simulink model "DAB Converters ude"  (R2022a)
settings: Solver=VariableStepAuto  StartTime=0.0  StopTime=0.7  RelTol=1e-3
libraries: spsMosfetLib x16, spsSeriesRLCBranchLib x8, spsCurrentMeasurementLib x4, spsLinearTransformerLib x4, simulink_extras x4, spsSawtoothGeneratorLib x4, spsVoltageMeasurementLib x4, spspowerguiLib x3, spsControlledVoltageSourceLib x2, spsIdealSwitchLib x2, slpidlib x1
settings Model: Creator=shuai  LastModifiedBy=shuai

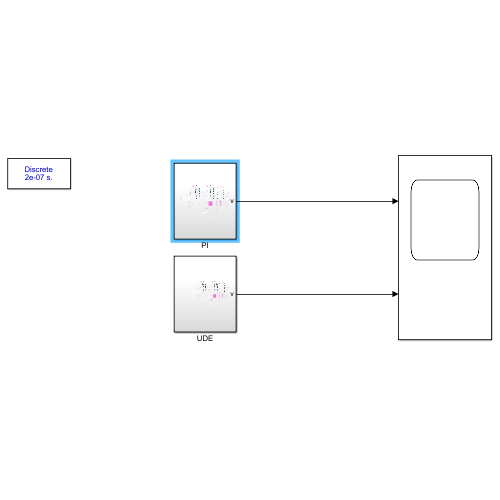
[thumbnail: Simulink's stored preview of the top-level diagram]
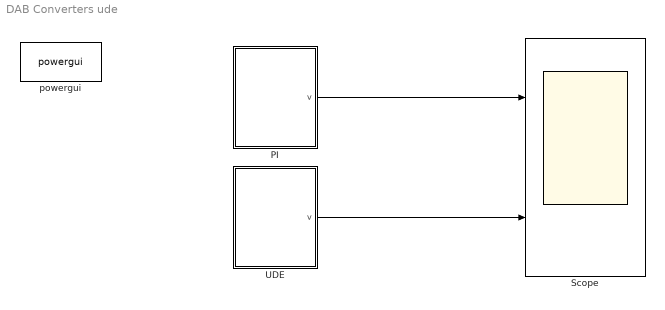
== system DAB Converters ude ==
  PI : Subsystem
  Scope : Scope  NumInputPorts=2
  UDE : Subsystem
  powergui : spspowerguiLib/powergui  Priority=1  SimulationMode=Discrete  SampleTime=2e-7  frequency=60  Iterations=50  frequencyindice=0  Pbase=100e6  ErrMax=1e-4  UnitsV=kV  UnitsW=MW  buscounter=0  FunctionMessages=off  echomessages=off  EnableUseOfTLC=off  CurrentSourceSwitches=off  DisableSnubberDevices=off  DisableRonSwitches=off  DisableVfSwitches=off  DisplayEquations=off  AutomaticDiscreteSolvers=off  SolverType=Tustin/Backward Euler (TBE)  Interpol=off  ExternalGateDelay=off  methode=off  Ts=100  x0status=blocks  SPID=on  SwTol=0  HookPort=off  NonlinearTolerance=1e-4  nMaxIteration=100  ContinueOnMaxIteration=off  RestoreLinks=warning  ResistiveCurrentMeasurement=off  Frange=[0:2:500]  Ylog=off  Xlog=on  ShowGrid=off  save=off  variable=ZData  structure=0  ZoomFFT=off  StartTime=0.0  cycles=1  DisplayStyle=1  fundamental=60  FreqAxis=off  MaxFrequency=1000  frequencyindicesteady=1  RmsSteady=1  display=off
  wires:
  UDE/1(v) -> Scope/2
  PI/1(v) -> Scope/1

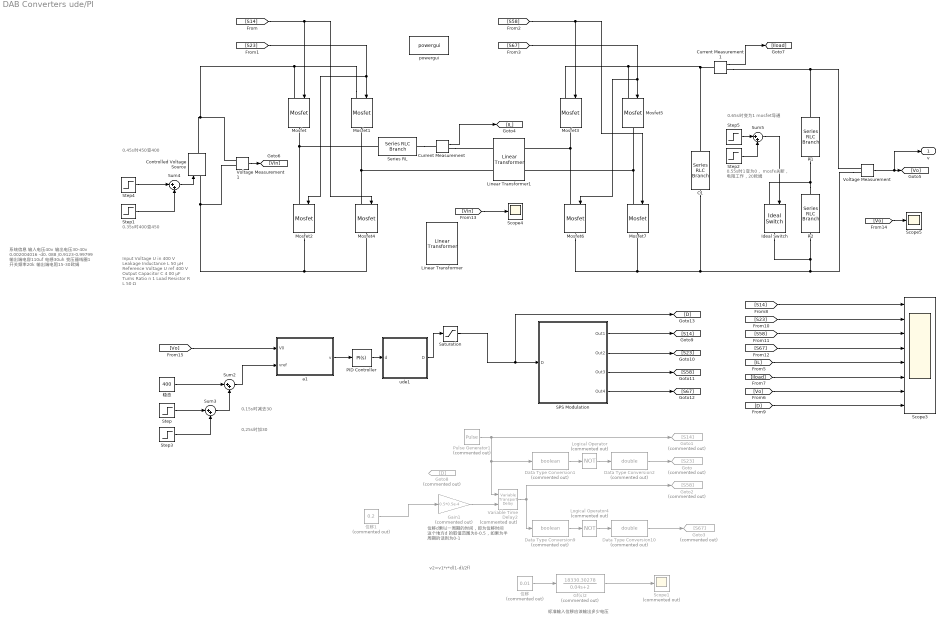
== system DAB Converters ude/PI ==
  note: 0.55s时1变为0，
      | mosfe关断，
      | 电阻工作，20欧姆
  note: 0.65s时变为1 mosfet导通
  note: 0.35s时400变450
  note: 0,15s时减去30
  note: 位移d乘以一周期的时间，即为位移时间
      | 这个地方d 的取值范围为0-0.5，如果为半
      | 周期的话则为0-1
  note: Input Voltage U in 400 V
      | Leakage Inductance L 50 µH
      | Reference Voltage U ref 400 V
      | Output Capacitor C 4 00 µF
      | Turns Ratio n 1
      | Load Resistor R L 50 Ω
  note: v2=v1*r*d(1-d)/2fl
  note: 系统信息
      | 输入电压40v
      | 输出电压30-40v
      | 0.002004016 -d0. 088 /0.9123-0.99799
      | 输出端电容110uf
      | 电感30uh
      | 变压器线圈1
      | 开关频率20k
      | 输出端电阻15-30欧姆
  note: 标准输入位移应该输出多少电压
  note: 0,25s时加30
  note: 0.45s时450变400
  C1 : spsSeriesRLCBranchLib/Series RLC Branch  LConnTagsString=__new0  RConnTagsString=__new0  BranchType=C  Resistance=0.01  Inductance=1e-3  SetiL0=off  InitialCurrent=0  Capacitance=400e-6  Setx0=on  InitialVoltage=0  Measurements=None
  Controlled Voltage Source : spsControlledVoltageSourceLib/Controlled Voltage Source  Initialize=on  Source_Type=DC  Amplitude=0  Phase=0  Frequency=0  Measurements=None
  Current Measurement : spsCurrentMeasurementLib/Current Measurement  PhasorSimulation=off  OutputType=Complex  PSBequivalent=0
  Current Measurement1 : spsCurrentMeasurementLib/Current Measurement  PhasorSimulation=off  OutputType=Complex  PSBequivalent=0
  Data Type Conversion1 : DataTypeConversion  Commented=on  OutDataTypeStr=boolean  SaturateOnIntegerOverflow=off  RndMeth=Floor
  Data Type Conversion10 : DataTypeConversion  Commented=on  OutDataTypeStr=double  SaturateOnIntegerOverflow=off  RndMeth=Floor
  Data Type Conversion2 : DataTypeConversion  Commented=on  OutDataTypeStr=double  SaturateOnIntegerOverflow=off  RndMeth=Floor
  Data Type Conversion9 : DataTypeConversion  Commented=on  OutDataTypeStr=boolean  SaturateOnIntegerOverflow=off  RndMeth=Floor
  Gain1 : Gain  Commented=on  Gain=0.5*0.5e-4
  Gf(s)2 : TransferFcn  Commented=on  Numerator=[18330.30278]  Denominator=[0.04 2]
  Goto : Goto  Commented=on  GotoTag=S23
  Goto1 : Goto  Commented=on  GotoTag=S14
  Goto2 : Goto  Commented=on  GotoTag=S58
  Goto3 : Goto  Commented=on  GotoTag=S67
  Goto8 : Goto  Commented=on  GotoTag=D
  Ideal Switch : spsIdealSwitchLib/Ideal Switch  Ron=0.001  Lon=0  IC=0  Rs=1e5  Cs=inf  Measurements=off
  Linear Transformer : spsLinearTransformerLib/Linear Transformer  UNITS=SI  NominalPower=[20e3 20000 ]  winding1=[500 0.0001 1e-08]  winding2=[500 0.0001 1e-08]  ThreeWindings=off  winding3=[3.15e+05 39690 12.634]  RmLm=[1e9 3439]  Measurements=None  DataType=on
  Linear Transformer1 : spsLinearTransformerLib/Linear Transformer  UNITS=SI  NominalPower=[20e5 20000 ]  winding1=[1000 0 0]  winding2=[1000 0 0]  ThreeWindings=off  winding3=[3.15e+05 39690 12.634]  RmLm=[8.5e4 8.5e4]  Measurements=None  DataType=on
  Logical Operator : Logic  Commented=on  Operator=NOT  AllPortsSameDT=off  OutDataTypeStr=boolean
  Logical Operator4 : Logic  Commented=on  Operator=NOT  AllPortsSameDT=off  OutDataTypeStr=boolean
  Mosfet{,1..7} (8 alike) : spsMosfetLib/Mosfet  Ron=0.001  Lon=0  Rd=0.001  Vfd=0  IC=0  Rs=1e5  Cs=inf  Measurements=off
  PID Controller : slpidlib/PID Controller  Controller=PI  Form=Parallel  TimeDomain=Continuous-time  UseExternalTs=off  SampleTime=-1  IntegratorMethod=Forward Euler  FilterMethod=Forward Euler  ControllerParametersSource=internal  P=0.000544489  I=0.116994  UseKiTs=off  D=0  N=100  UseFilter=on  TunerSelectOption=Transfer Function Based (PID Tuner App)  InitialConditionSource=internal  InitialConditionForIntegrator=0  InitialConditionForFilter=0  DifferentiatorICPrevScaledInput=0  ExternalReset=none  TrackingMode=off  Kt=1  LimitOutput=off  SatLimitsSource=internal  UpperSaturationLimit=inf  LowerSaturationLimit=-inf  LinearizeAsGain=on  AntiWindupMode=none  Kb=1  POutMin=[]  POutMax=[]  IOutMin=[]  IOutMax=[]  DOutMin=[]  DOutMax=[]  NOutMin=[]  NOutMax=[]  SumOutMin=[]  SumOutMax=[]  SaturationOutMin=[]  SaturationOutMax=[]  PParamMin=[]  PParamMax=[]  IParamMin=[]  IParamMax=[]  DParamMin=[]  DParamMax=[]  NParamMin=[]  NParamMax=[]  KbParamMin=[]  KbParamMax=[]  KtParamMin=[]  KtParamMax=[]  KbOutMin=[]  KbOutMax=[]  KtOutMin=[]  KtOutMax=[]  IntegratorOutMin=[]  IntegratorOutMax=[]  FilterOutMin=[]  FilterOutMax=[]  SumI1OutMin=[]  SumI1OutMax=[]  SumI2OutMin=[]  SumI2OutMax=[]  SumI3OutMin=[]  SumI3OutMax=[]  SumI4OutMin=[]  SumI4OutMax=[]  SumDOutMin=[]  SumDOutMax=[]  DifferentiatorOutMin=[]  DifferentiatorOutMax=[]  FilterDiffOutCoefMin=[]  FilterDiffOutCoefMax=[]  ReciprocalOutMin=[]  ReciprocalOutMax=[]  SumDenOutMin=[]  SumDenOutMax=[]  SumNumOutMin=[]  SumNumOutMax=[]  DivideOutMin=[]  DivideOutMax=[]  UdiffTsProdOutMin=[]  UdiffTsProdOutMax=[]  NTsProdOutMin=[]  NTsProdOutMax=[]  UintegralTsProdOutMin=[]  UintegralTsProdOutMax=[]  UngainTsProdOutMin=[]  UngainTsProdOutMax=[]  IntegratorContinuousStateAttributes=''  IntegratorStateMustResolveToSignalObject=off  IntegratorRTWStateStorageClass=Auto  FilterContinuousStateAttributes=''  FilterStateMustResolveToSignalObject=off  FilterRTWStateStorageClass=Auto  ParallelPVariant=InternalParameters  IdealPVariant=Disabled  IVariant=InternalParameters  DVariant=Disabled  IntegratorVariant=Continuous  SatVariant=Disabled  AWVariant=Passthrough  PCopyVariant=Disabled  TRVariant=Disabled  FdbkBlocksVariant=Forward  IdealPFdbkVariant=Disabled  SatFdbkVariant=Disabled  DerivativeFilterVariant=Disabled  NVariant=Disabled  NCopyVariant=Disabled_SignalSpec  FilterICVariant=Disabled  IntegratorICVariant=InternalICs  ExternalResetVariant=Disabled  TRSumVariant=Passthrough  SumFdbkVariant=Disabled  SumVariant=Sum_PI  TsampFilterVariant=InternalTs  TsampNgainVariant=Passthrough  TsampIntegralVariant=Passthrough  ExternalSaturationOutDataTypeStr=Inherit: Same as second input  aMode=0
  Pulse Generator1 : DiscretePulseGenerator  Commented=on  PulseType=Time based  Period=1/20e3  PulseWidth=50
  R1 : spsSeriesRLCBranchLib/Series RLC Branch  LConnTagsString=__new0  RConnTagsString=__new0  BranchType=R  Resistance=50  Inductance=1e-3  SetiL0=off  InitialCurrent=0  Capacitance=1e-6  Setx0=off  InitialVoltage=0  Measurements=None
  R2 : spsSeriesRLCBranchLib/Series RLC Branch  LConnTagsString=__new0  RConnTagsString=__new0  BranchType=R  Resistance=10  Inductance=1e-3  SetiL0=off  InitialCurrent=0  Capacitance=1e-6  Setx0=off  InitialVoltage=0  Measurements=None
  SPS Modulation : Subsystem
  Saturation : Saturate  UpperLimit=0.9  LowerLimit=0
  Scope1 : Scope  Commented=on
  Scope3 : Scope  NumInputPorts=8
  Scope4 : Scope
  Scope5 : Scope
  Series RL : spsSeriesRLCBranchLib/Series RLC Branch  LConnTagsString=__new0  RConnTagsString=__new0  BranchType=RL  Resistance=0  Inductance=50e-6  SetiL0=off  InitialCurrent=0  Capacitance=1e-6  Setx0=off  InitialVoltage=0  Measurements=None
  Step : Step  Time=0.1  After=-30  SampleTime=0
  Step1 : Step  Time=0.3  Before=400  After=450  SampleTime=0
  Step2 : Step  Time=0.5  Before=1  After=0  SampleTime=0
  Step3 : Step  Time=0.2  After=50  SampleTime=0
  Step4 : Step  Time=0.4  After=-50  SampleTime=0
  Step5 : Step  Time=0.6  SampleTime=0
  Sum{2..5} (4 alike) : Sum  Inputs=|++
  Variable Time Delay2 : VariableTransportDelay  Commented=on  MaximumDelay=10  MaximumPoints=1024000  ZeroDelay=on
  Voltage Measurement : spsVoltageMeasurementLib/Voltage Measurement  PhasorSimulation=off  OutputType=Complex  PSBequivalent=0
  Voltage Measurement1 : spsVoltageMeasurementLib/Voltage Measurement  PhasorSimulation=off  OutputType=Complex  PSBequivalent=0
  a1 : MATLAB Function  TreatAsAtomicUnit=on  SystemSampleTime=1/20000
  powergui : spspowerguiLib/powergui  Priority=1  SimulationMode=Discrete  SampleTime=2e-7  frequency=60  Iterations=50  frequencyindice=0  Pbase=100e6  ErrMax=1e-4  UnitsV=kV  UnitsW=MW  buscounter=0  FunctionMessages=off  echomessages=off  EnableUseOfTLC=off  CurrentSourceSwitches=off  DisableSnubberDevices=off  DisableRonSwitches=off  DisableVfSwitches=off  DisplayEquations=off  AutomaticDiscreteSolvers=off  SolverType=Tustin/Backward Euler (TBE)  Interpol=off  ExternalGateDelay=off  methode=off  Ts=100  x0status=blocks  SPID=off  SwTol=0  HookPort=off  NonlinearTolerance=1e-4  nMaxIteration=100  ContinueOnMaxIteration=off  RestoreLinks=warning  ResistiveCurrentMeasurement=off  Frange=[0:2:500]  Ylog=off  Xlog=on  ShowGrid=off  save=off  variable=ZData  structure=0  ZoomFFT=off  StartTime=0.0  cycles=1  DisplayStyle=1  fundamental=60  FreqAxis=off  MaxFrequency=1000  frequencyindicesteady=1  RmsSteady=1  display=off
  ude1 : MATLAB Function  TreatAsAtomicUnit=on  SystemSampleTime=1/20000
  位移 : Constant  Commented=on  Value=0.01  VectorParams1D=off
  位移1 : Constant  Commented=on  Value=0.2  VectorParams1D=off
  稳态 : Constant  Value=400  VectorParams1D=off
  v : Outport
  wires:
  Variable Time Delay2/1 -> Goto2/1, Data Type Conversion9/1
  Gain1/1 -> Variable Time Delay2/2
  SPS Modulation/4(Out4) -> [S67]
  Logical Operator4/1 -> Data Type Conversion10/1
  [S23] -> Scope3/2
  Current Measurement1/1 -> [Iload]
  [S67] -> Mosfet6/1, Mosfet5/1
  Data Type Conversion10/1 -> Goto3/1
  SPS Modulation/3(Out3) -> [S58]
  [S58] -> Mosfet7/1, Mosfet3/1
  Data Type Conversion9/1 -> Logical Operator4/1
  [S14] -> Scope3/1
  [Vin] -> Scope4/1
  Current Measurement/1 -> [IL]
  Sum4/1 -> Controlled Voltage Source/1
  [D] -> Scope3/8
  Data Type Conversion2/1 -> Goto/1
  稳态/1 -> Sum2/1
  Sum2/1 -> a1/2(vref)
  Step4/1 -> Sum4/1
  Voltage Measurement1/1 -> [Vin]
  Data Type Conversion1/1 -> Logical Operator/1
  位移/1 -> Gf(s)2/1
  Gf(s)2/1 -> Scope1/1
  Step5/1 -> Sum5/1
  [Vo] -> Scope5/1
  Saturation/1 -> [D], SPS Modulation/1(D)
  Pulse Generator1/1 -> Goto1/1, Data Type Conversion1/1, Variable Time Delay2/1
  [S23] -> Mosfet2/1, Mosfet1/1
  Step/1 -> Sum3/1
  Voltage Measurement/1 -> v/1, [Vo]
  SPS Modulation/2(Out2) -> [S23]
  [S14] -> Mosfet4/1, Mosfet/1
  Logical Operator/1 -> Data Type Conversion2/1
  SPS Modulation/1(Out1) -> [S14]
  [S67] -> Scope3/4
  [Iload] -> Scope3/6
  [S58] -> Scope3/3
  Step1/1 -> Sum4/2
  Sum3/1 -> Sum2/2
  位移1/1 -> Gain1/1
  Step3/1 -> Sum3/2
  [IL] -> Scope3/5
  Sum5/1 -> Ideal Switch/1
  Step2/1 -> Sum5/2
  [Vo] -> Scope3/7
  ude1/1(D) -> Saturation/1
  a1/1(v) -> PID Controller/1
  PID Controller/1 -> ude1/1(d)
  [Vo] -> a1/1(V0)
  connections:
  Mosfet1/LConn1 -- Voltage Measurement1/LConn1 -- Controlled Voltage Source/RConn1 -- Mosfet/LConn1
  Mosfet4/RConn1 -- Voltage Measurement1/LConn2 -- Controlled Voltage Source/LConn1 -- Mosfet2/RConn1
  Linear Transformer1/RConn2 -- Mosfet7/LConn1 -- Mosfet5/RConn1
  Current Measurement1/LConn1 -- C1/LConn1 -- Mosfet5/LConn1 -- Mosfet3/LConn1
  Current Measurement1/RConn1 -- R1/LConn1 -- Voltage Measurement/LConn1
  Voltage Measurement/LConn2 -- C1/RConn1 -- Mosfet6/RConn1 -- Mosfet7/RConn1 -- Ideal Switch/RConn1 -- R2/RConn1
  Series RL/RConn1 -- Current Measurement/LConn1
  R2/LConn1 -- R1/RConn1 -- Ideal Switch/LConn1
  Series RL/LConn1 -- Mosfet/RConn1 -- Mosfet2/LConn1
  Mosfet1/RConn1 -- Mosfet4/LConn1 -- Linear Transformer1/LConn2
  Current Measurement/RConn1 -- Linear Transformer1/LConn1
  Linear Transformer1/RConn1 -- Mosfet6/LConn1 -- Mosfet3/RConn1

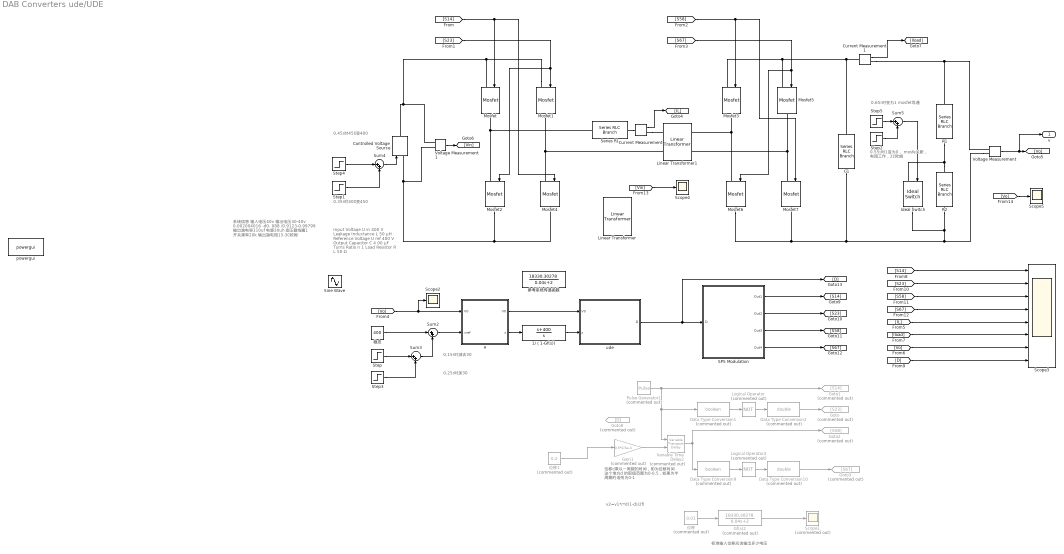
== system DAB Converters ude/UDE ==
  note: 0.55s时1变为0，
      | mosfe关断，
      | 电阻工作，20欧姆
  note: 0.65s时变为1 mosfet导通
  note: 0.35s时400变450
  note: 0,15s时减去30
  note: 位移d乘以一周期的时间，即为位移时间
      | 这个地方d 的取值范围为0-0.5，如果为半
      | 周期的话则为0-1
  note: Input Voltage U in 400 V
      | Leakage Inductance L 50 µH
      | Reference Voltage U ref 400 V
      | Output Capacitor C 4 00 µF
      | Turns Ratio n 1
      | Load Resistor R L 50 Ω
  note: v2=v1*r*d(1-d)/2fl
  note: 系统信息
      | 输入电压40v
      | 输出电压30-40v
      | 0.002004016 -d0. 088 /0.9123-0.99799
      | 输出端电容110uf
      | 电感30uh
      | 变压器线圈1
      | 开关频率20k
      | 输出端电阻15-30欧姆
  note: 标准输入位移应该输出多少电压
  note: 0,25s时加30
  note: 0.45s时450变400
  1/（1-Gf(s)) : TransferFcn  Numerator=[1 400]  Denominator=[1 0]
  C1 : spsSeriesRLCBranchLib/Series RLC Branch  LConnTagsString=__new0  RConnTagsString=__new0  BranchType=C  Resistance=0.01  Inductance=1e-3  SetiL0=off  InitialCurrent=0  Capacitance=400e-6  Setx0=on  InitialVoltage=0  Measurements=None
  Controlled Voltage Source : spsControlledVoltageSourceLib/Controlled Voltage Source  Initialize=on  Source_Type=DC  Amplitude=0  Phase=0  Frequency=0  Measurements=None
  Current Measurement : spsCurrentMeasurementLib/Current Measurement  PhasorSimulation=off  OutputType=Complex  PSBequivalent=0
  Current Measurement1 : spsCurrentMeasurementLib/Current Measurement  PhasorSimulation=off  OutputType=Complex  PSBequivalent=0
  Data Type Conversion1 : DataTypeConversion  Commented=on  OutDataTypeStr=boolean  SaturateOnIntegerOverflow=off  RndMeth=Floor
  Data Type Conversion10 : DataTypeConversion  Commented=on  OutDataTypeStr=double  SaturateOnIntegerOverflow=off  RndMeth=Floor
  Data Type Conversion2 : DataTypeConversion  Commented=on  OutDataTypeStr=double  SaturateOnIntegerOverflow=off  RndMeth=Floor
  Data Type Conversion9 : DataTypeConversion  Commented=on  OutDataTypeStr=boolean  SaturateOnIntegerOverflow=off  RndMeth=Floor
  Gain1 : Gain  Commented=on  Gain=0.5*0.5e-4
  Gf(s)2 : TransferFcn  Commented=on  Numerator=[18330.30278]  Denominator=[0.04 2]
  Goto : Goto  Commented=on  GotoTag=S23
  Goto1 : Goto  Commented=on  GotoTag=S14
  Goto2 : Goto  Commented=on  GotoTag=S58
  Goto3 : Goto  Commented=on  GotoTag=S67
  Goto8 : Goto  Commented=on  GotoTag=D
  Ideal Switch : spsIdealSwitchLib/Ideal Switch  Ron=0.001  Lon=0  IC=0  Rs=1e5  Cs=inf  Measurements=off
  Linear Transformer : spsLinearTransformerLib/Linear Transformer  UNITS=SI  NominalPower=[20e3 20000 ]  winding1=[500 0.0001 1e-08]  winding2=[500 0.0001 1e-08]  ThreeWindings=off  winding3=[3.15e+05 39690 12.634]  RmLm=[1e9 3439]  Measurements=None  DataType=on
  Linear Transformer1 : spsLinearTransformerLib/Linear Transformer  UNITS=SI  NominalPower=[20e5 20000 ]  winding1=[1000 0 0]  winding2=[1000 0 0]  ThreeWindings=off  winding3=[3.15e+05 39690 12.634]  RmLm=[8.5e4 8.5e4]  Measurements=None  DataType=on
  Logical Operator : Logic  Commented=on  Operator=NOT  AllPortsSameDT=off  OutDataTypeStr=boolean
  Logical Operator4 : Logic  Commented=on  Operator=NOT  AllPortsSameDT=off  OutDataTypeStr=boolean
  Mosfet{,1..7} (8 alike) : spsMosfetLib/Mosfet  Ron=0.001  Lon=0  Rd=0.001  Vfd=0  IC=0  Rs=1e5  Cs=inf  Measurements=off
  Pulse Generator1 : DiscretePulseGenerator  Commented=on  PulseType=Time based  Period=1/20e3  PulseWidth=50
  R1 : spsSeriesRLCBranchLib/Series RLC Branch  LConnTagsString=__new0  RConnTagsString=__new0  BranchType=R  Resistance=50  Inductance=1e-3  SetiL0=off  InitialCurrent=0  Capacitance=1e-6  Setx0=off  InitialVoltage=0  Measurements=None
  R2 : spsSeriesRLCBranchLib/Series RLC Branch  LConnTagsString=__new0  RConnTagsString=__new0  BranchType=R  Resistance=10  Inductance=1e-3  SetiL0=off  InitialCurrent=0  Capacitance=1e-6  Setx0=off  InitialVoltage=0  Measurements=None
  SPS Modulation : Subsystem
  Scope1 : Scope  Commented=on
  Scope2 : Scope
  Scope3 : Scope  NumInputPorts=8
  Scope4 : Scope
  Scope5 : Scope
  Series RL : spsSeriesRLCBranchLib/Series RLC Branch  LConnTagsString=__new0  RConnTagsString=__new0  BranchType=L  Resistance=0  Inductance=50e-6  SetiL0=off  InitialCurrent=0  Capacitance=1e-6  Setx0=off  InitialVoltage=0  Measurements=None
  Sine Wave : Sin  Amplitude=10  Frequency=1000  SampleTime=0
  Step : Step  Time=0.1  After=-30  SampleTime=0
  Step1 : Step  Time=0.3  Before=400  After=450  SampleTime=0
  Step2 : Step  Time=0.5  Before=1  After=0  SampleTime=0
  Step3 : Step  Time=0.2  After=50  SampleTime=0
  Step4 : Step  Time=0.4  After=-50  SampleTime=0
  Step5 : Step  Time=0.6  SampleTime=0
  Sum{2..5} (4 alike) : Sum  Inputs=|++
  Variable Time Delay2 : VariableTransportDelay  Commented=on  MaximumDelay=10  MaximumPoints=1024000  ZeroDelay=on
  Voltage Measurement : spsVoltageMeasurementLib/Voltage Measurement  PhasorSimulation=off  OutputType=Complex  PSBequivalent=0
  Voltage Measurement1 : spsVoltageMeasurementLib/Voltage Measurement  PhasorSimulation=off  OutputType=Complex  PSBequivalent=0
  a : MATLAB Function  TreatAsAtomicUnit=on  SystemSampleTime=1/20000
  powergui : spspowerguiLib/powergui  Priority=1  SimulationMode=Discrete  SampleTime=2e-7  frequency=60  Iterations=50  frequencyindice=0  Pbase=100e6  ErrMax=1e-4  UnitsV=kV  UnitsW=MW  buscounter=0  FunctionMessages=off  echomessages=off  EnableUseOfTLC=off  CurrentSourceSwitches=off  DisableSnubberDevices=off  DisableRonSwitches=off  DisableVfSwitches=off  DisplayEquations=off  AutomaticDiscreteSolvers=off  SolverType=Tustin/Backward Euler (TBE)  Interpol=off  ExternalGateDelay=off  methode=off  Ts=100  x0status=blocks  SPID=off  SwTol=0  HookPort=off  NonlinearTolerance=1e-4  nMaxIteration=100  ContinueOnMaxIteration=off  RestoreLinks=warning  ResistiveCurrentMeasurement=off  Frange=[0:2:500]  Ylog=off  Xlog=on  ShowGrid=off  save=off  variable=ZData  structure=0  ZoomFFT=off  StartTime=0.0  cycles=1  DisplayStyle=1  fundamental=60  FreqAxis=off  MaxFrequency=1000  frequencyindicesteady=1  RmsSteady=1  display=off
  ude : MATLAB Function  TreatAsAtomicUnit=on  SystemSampleTime=1/20000
  位移 : Constant  Commented=on  Value=0.01  VectorParams1D=off
  位移1 : Constant  Commented=on  Value=0.2  VectorParams1D=off
  参考系统传递函数 : TransferFcn  Numerator=[18330.30278]  Denominator=[0.04 2]
  稳态 : Constant  Value=400  VectorParams1D=off
  v : Outport
  wires:
  Variable Time Delay2/1 -> Goto2/1, Data Type Conversion9/1
  Gain1/1 -> Variable Time Delay2/2
  SPS Modulation/4(Out4) -> [S67]
  Logical Operator4/1 -> Data Type Conversion10/1
  [S23] -> Scope3/2
  Current Measurement1/1 -> [Iload]
  [S67] -> Mosfet6/1, Mosfet5/1
  Data Type Conversion10/1 -> Goto3/1
  SPS Modulation/3(Out3) -> [S58]
  [S58] -> Mosfet7/1, Mosfet3/1
  Data Type Conversion9/1 -> Logical Operator4/1
  [S14] -> Scope3/1
  [Vin] -> Scope4/1
  Current Measurement/1 -> [IL]
  Sum4/1 -> Controlled Voltage Source/1
  [D] -> Scope3/8
  1/（1-Gf(s))/1 -> ude/2(z)
  Data Type Conversion2/1 -> Goto/1
  稳态/1 -> Sum2/1
  Sum2/1 -> a/2(vref)
  Step4/1 -> Sum4/1
  Voltage Measurement1/1 -> [Vin]
  Data Type Conversion1/1 -> Logical Operator/1
  位移/1 -> Gf(s)2/1
  Gf(s)2/1 -> Scope1/1
  Step5/1 -> Sum5/1
  [Vo] -> Scope5/1
  ude/1(D) -> [D], SPS Modulation/1(D)
  Pulse Generator1/1 -> Goto1/1, Data Type Conversion1/1, Variable Time Delay2/1
  [S23] -> Mosfet2/1, Mosfet1/1
  a/1(V0) -> ude/1(V0)
  Step/1 -> Sum3/1
  Voltage Measurement/1 -> v/1, [Vo]
  a/2(z) -> 1/（1-Gf(s))/1
  SPS Modulation/2(Out2) -> [S23]
  [S14] -> Mosfet4/1, Mosfet/1
  Logical Operator/1 -> Data Type Conversion2/1
  SPS Modulation/1(Out1) -> [S14]
  [S67] -> Scope3/4
  [Iload] -> Scope3/6
  [S58] -> Scope3/3
  Step1/1 -> Sum4/2
  [Vo] -> a/1("V0 "), Scope2/1
  Sum3/1 -> Sum2/2
  位移1/1 -> Gain1/1
  Step3/1 -> Sum3/2
  [IL] -> Scope3/5
  Sum5/1 -> Ideal Switch/1
  Step2/1 -> Sum5/2
  [Vo] -> Scope3/7
  connections:
  Mosfet1/LConn1 -- Voltage Measurement1/LConn1 -- Controlled Voltage Source/RConn1 -- Mosfet/LConn1
  Mosfet4/RConn1 -- Voltage Measurement1/LConn2 -- Controlled Voltage Source/LConn1 -- Mosfet2/RConn1
  Linear Transformer1/RConn2 -- Mosfet7/LConn1 -- Mosfet5/RConn1
  Current Measurement1/LConn1 -- C1/LConn1 -- Mosfet5/LConn1 -- Mosfet3/LConn1
  Current Measurement1/RConn1 -- R1/LConn1 -- Voltage Measurement/LConn1
  Voltage Measurement/LConn2 -- C1/RConn1 -- Mosfet6/RConn1 -- Mosfet7/RConn1 -- Ideal Switch/RConn1 -- R2/RConn1
  Series RL/RConn1 -- Current Measurement/LConn1
  R2/LConn1 -- R1/RConn1 -- Ideal Switch/LConn1
  Mosfet1/RConn1 -- Mosfet4/LConn1 -- Linear Transformer1/LConn2
  Current Measurement/RConn1 -- Linear Transformer1/LConn1
  Linear Transformer1/RConn1 -- Mosfet6/LConn1 -- Mosfet3/RConn1
  Mosfet2/LConn1 -- Series RL/LConn1 -- Mosfet/RConn1

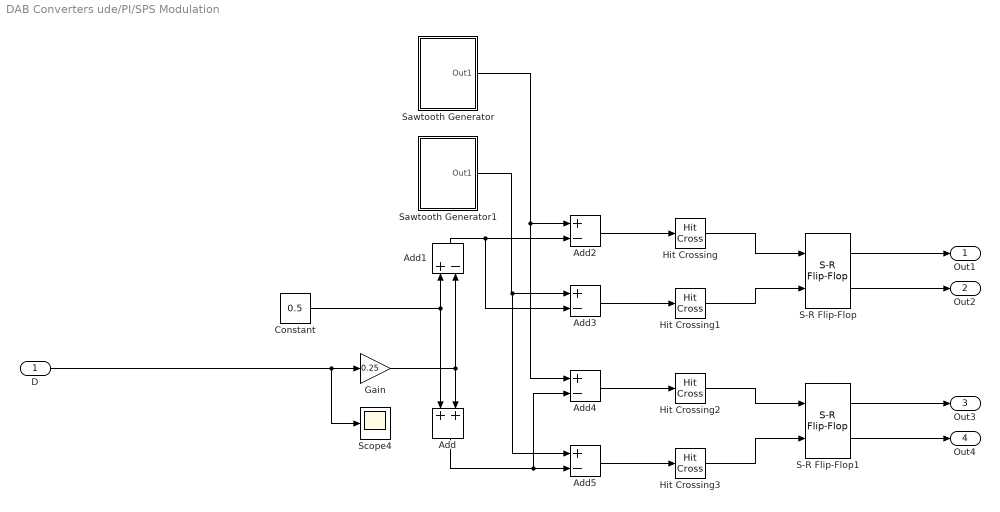
== system DAB Converters ude/PI/SPS Modulation ==
  D : Inport
  Add : Sum
  Add{1..5} (5 alike) : Sum  Inputs=+-
  Constant : Constant  Value=0.5
  Gain : Gain  Gain=0.25
  Hit Crossing{,1..3} (4 alike) : HitCross  HitCrossingDirection=rising
  S-R Flip-Flop : simulink_extras/Flip Flops/S-R Flip-Flop  initial_condition=0
  S-R Flip-Flop1 : simulink_extras/Flip Flops/S-R Flip-Flop  initial_condition=0
  Sawtooth Generator : Subsystem  mask{fs=20000}
      mask prompts: fs "Frequency (Hz)"
      mask help: Sawtooth Generator
  Sawtooth Generator1 : Subsystem  mask{fs=20000}
      mask prompts: fs "Frequency (Hz)"
      mask help: Sawtooth Generator
  Scope4 : Scope
  Out1 : Outport  VectorParamsAs1DForOutWhenUnconnected=off
  Out2 : Outport  Port=2  VectorParamsAs1DForOutWhenUnconnected=off
  Out3 : Outport  Port=3  VectorParamsAs1DForOutWhenUnconnected=off
  Out4 : Outport  Port=4  VectorParamsAs1DForOutWhenUnconnected=off
  wires:
  Hit Crossing1/1 -> S-R Flip-Flop/2
  Add1/1 -> Add3/2, Add2/2
  Constant/1 -> Add1/1, Add/1
  Add5/1 -> Hit Crossing3/1
  Gain/1 -> Add1/2, Add/2
  D/1 -> Gain/1, Scope4/1
  Add/1 -> Add4/2, Add5/2
  Sawtooth Generator/1(Out1) -> Add4/1, Add2/1
  Hit Crossing/1 -> S-R Flip-Flop/1
  Add2/1 -> Hit Crossing/1
  Sawtooth Generator1/1(Out1) -> Add5/1, Add3/1
  Add3/1 -> Hit Crossing1/1
  Add4/1 -> Hit Crossing2/1
  Hit Crossing2/1 -> S-R Flip-Flop1/1
  Hit Crossing3/1 -> S-R Flip-Flop1/2
  S-R Flip-Flop1/1 -> Out3/1
  S-R Flip-Flop1/2 -> Out4/1
  S-R Flip-Flop/1 -> Out1/1
  S-R Flip-Flop/2 -> Out2/1

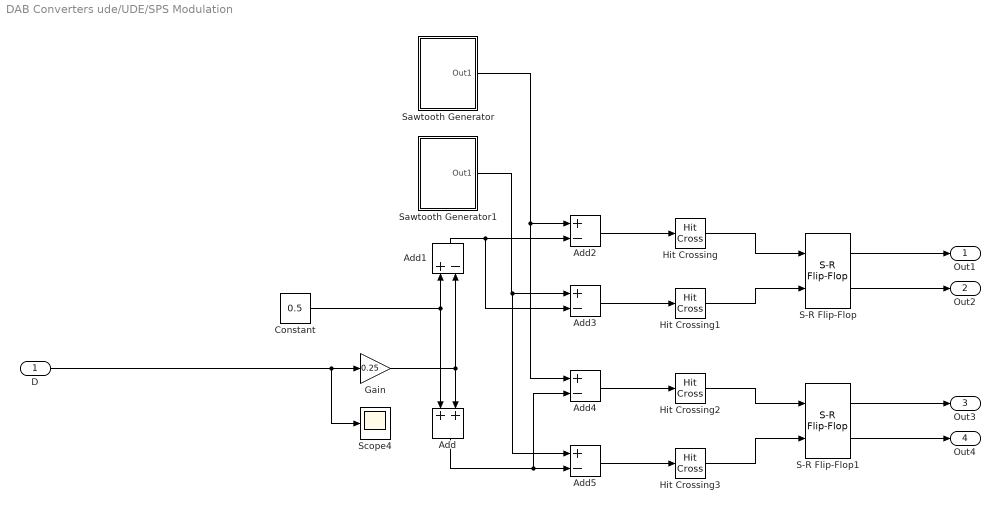
== system DAB Converters ude/UDE/SPS Modulation ==
  D : Inport
  Add : Sum
  Add{1..5} (5 alike) : Sum  Inputs=+-
  Constant : Constant  Value=0.5
  Gain : Gain  Gain=0.25
  Hit Crossing{,1..3} (4 alike) : HitCross  HitCrossingDirection=rising
  S-R Flip-Flop : simulink_extras/Flip Flops/S-R Flip-Flop  initial_condition=0
  S-R Flip-Flop1 : simulink_extras/Flip Flops/S-R Flip-Flop  initial_condition=0
  Sawtooth Generator : Subsystem  mask{fs=20000}
      mask prompts: fs "Frequency (Hz)"
      mask help: Sawtooth Generator
  Sawtooth Generator1 : Subsystem  mask{fs=20000}
      mask prompts: fs "Frequency (Hz)"
      mask help: Sawtooth Generator
  Scope4 : Scope
  Out1 : Outport  VectorParamsAs1DForOutWhenUnconnected=off
  Out2 : Outport  Port=2  VectorParamsAs1DForOutWhenUnconnected=off
  Out3 : Outport  Port=3  VectorParamsAs1DForOutWhenUnconnected=off
  Out4 : Outport  Port=4  VectorParamsAs1DForOutWhenUnconnected=off
  wires:
  Hit Crossing1/1 -> S-R Flip-Flop/2
  Add1/1 -> Add3/2, Add2/2
  Constant/1 -> Add1/1, Add/1
  Add5/1 -> Hit Crossing3/1
  Gain/1 -> Add1/2, Add/2
  D/1 -> Gain/1, Scope4/1
  Add/1 -> Add4/2, Add5/2
  Sawtooth Generator/1(Out1) -> Add4/1, Add2/1
  Hit Crossing/1 -> S-R Flip-Flop/1
  Add2/1 -> Hit Crossing/1
  Sawtooth Generator1/1(Out1) -> Add5/1, Add3/1
  Add3/1 -> Hit Crossing1/1
  Add4/1 -> Hit Crossing2/1
  Hit Crossing2/1 -> S-R Flip-Flop1/1
  Hit Crossing3/1 -> S-R Flip-Flop1/2
  S-R Flip-Flop1/1 -> Out3/1
  S-R Flip-Flop1/2 -> Out4/1
  S-R Flip-Flop/1 -> Out1/1
  S-R Flip-Flop/2 -> Out2/1

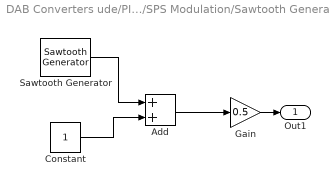
== system DAB Converters ude/PI/SPS Modulation/Sawtooth Generator ==
  Add : Sum
  Constant : Constant
  Gain : Gain  Gain=0.5
  Sawtooth Generator : spsSawtoothGeneratorLib/Sawtooth Generator  Freq=fs  Phase=180  Ts=0
  Out1 : Outport  VectorParamsAs1DForOutWhenUnconnected=off
  wires:
  Add/1 -> Gain/1
  Gain/1 -> Out1/1
  Constant/1 -> Add/2
  Sawtooth Generator/1 -> Add/1

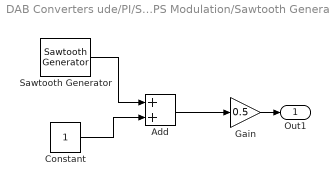
== system DAB Converters ude/PI/SPS Modulation/Sawtooth Generator1 ==
  Add : Sum
  Constant : Constant
  Gain : Gain  Gain=0.5
  Sawtooth Generator : spsSawtoothGeneratorLib/Sawtooth Generator  Freq=fs  Phase=0  Ts=0
  Out1 : Outport  VectorParamsAs1DForOutWhenUnconnected=off
  wires:
  Add/1 -> Gain/1
  Gain/1 -> Out1/1
  Constant/1 -> Add/2
  Sawtooth Generator/1 -> Add/1

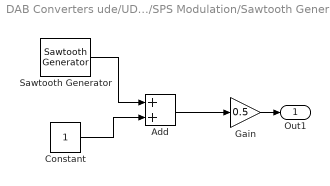
== system DAB Converters ude/UDE/SPS Modulation/Sawtooth Generator ==
  Add : Sum
  Constant : Constant
  Gain : Gain  Gain=0.5
  Sawtooth Generator : spsSawtoothGeneratorLib/Sawtooth Generator  Freq=fs  Phase=180  Ts=0
  Out1 : Outport  VectorParamsAs1DForOutWhenUnconnected=off
  wires:
  Add/1 -> Gain/1
  Gain/1 -> Out1/1
  Constant/1 -> Add/2
  Sawtooth Generator/1 -> Add/1

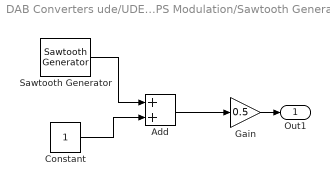
== system DAB Converters ude/UDE/SPS Modulation/Sawtooth Generator1 ==
  Add : Sum
  Constant : Constant
  Gain : Gain  Gain=0.5
  Sawtooth Generator : spsSawtoothGeneratorLib/Sawtooth Generator  Freq=fs  Phase=0  Ts=0
  Out1 : Outport  VectorParamsAs1DForOutWhenUnconnected=off
  wires:
  Add/1 -> Gain/1
  Gain/1 -> Out1/1
  Constant/1 -> Add/2
  Sawtooth Generator/1 -> Add/1

== matlab function DAB Converters ude/UDE/a ==
  data: V0 output; V0 input; z output; vref input
function [V0,z] = fcn(V0,vref)

Am=-400;%%Xm点=-αXm(t)+-αC(t)
Bm=400;%%
k=0;
vowen=400;
v=V0-vowen;
c=vref-vowen;%%c为相较于稳态时期望电压的变化值
e=c-v;
z=Am*v+Bm*c-k*e;

== matlab function DAB Converters ude/UDE/ude ==
  data: V0 input; D output; z input
function D = fcn(V0,z)
fs=20e3;%%工作频率
n=1;
C=400e-6;%%输出端电容
L=50e-6;%%电感
V1=400;%%输入电压
R=50;%%输出端电压
D1=0.5-0.1*sqrt(21);%%当输出电压为400v时，根据输处电压与输入d之间的关系求得
A=-1/(R*C);
B=n*(1-2*D1)*V1/(2*fs*L*C);%%小信号建模后，D1为稳态值时输出电压
vowen=400;
beita=400;%%   Gf（s）= β/(s+β) 中的β
v=V0-vowen;%% v为电压相对于第一次稳态时的变压变化，vowen为第一次稳态的电压，Vo为输出电压
d=(-1/B)*(A*v+v*beita-z);%%z
D=D1+d;

== matlab function DAB Converters ude/PI/a1 ==
  data: V0 input; v output; vref input
function v = fcn(V0,vref)

vowen=400;
ve=V0-vowen;
c=vref-vowen;%%c为相较于稳态时期望电压的变化值
v=c-ve;

== matlab function DAB Converters ude/PI/ude1 ==
  data: d input; D output
function D = fcn(d)
D1=0.5-0.1*sqrt(21);
D=D1+d;
